simulink model "model_2022b"  (R2023b)
settings: Solver=VariableStepAuto  StartTime=0.0  StopTime=250  FixedStep=0.001  MaxStep=1e-2  RelTol=1e-3
undefined symbols (not defined in the file or in its folder): A, A0f, b, d, gamma, N, P
settings Model: Creator=Катя  LastModifiedBy=deniskirbaba

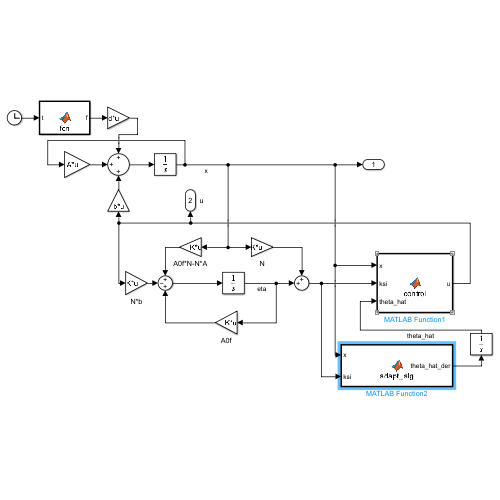
[thumbnail: Simulink's stored preview of the top-level diagram]
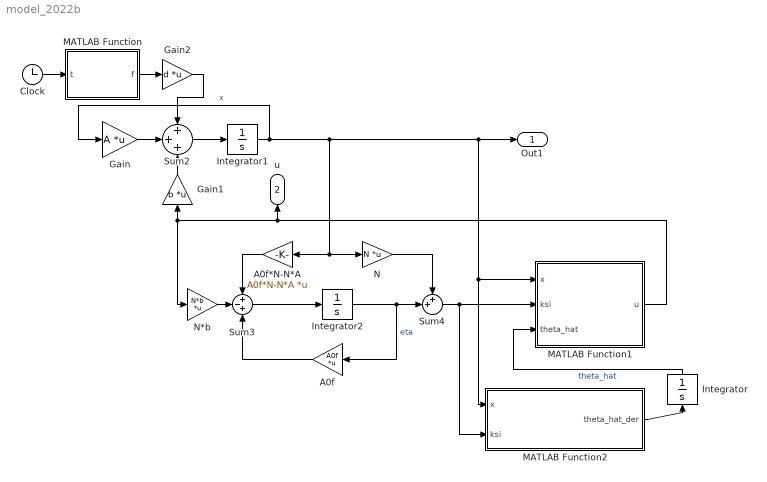
== system model_2022b ==
  A0f : Gain  Gain=A0f  Multiplication=Matrix(K*u)
  A0f*N-N*A : Gain  Gain=A0f*N-N*A  Multiplication=Matrix(K*u)
  Clock : Clock
  Gain : Gain  Gain=A  Multiplication=Matrix(K*u)
  Gain1 : Gain  Gain=b  Multiplication=Matrix(K*u)
  Gain2 : Gain  Gain=d  Multiplication=Matrix(K*u)
  Integrator : Integrator  InitialCondition=[0;0]
  Integrator1 : Integrator  InitialCondition=[0;0]
  Integrator2 : Integrator
  MATLAB Function : MATLAB Function  TreatAsAtomicUnit=on
  MATLAB Function1 : MATLAB Function  TreatAsAtomicUnit=on
  MATLAB Function2 : MATLAB Function  TreatAsAtomicUnit=on
  N : Gain  Gain=N  Multiplication=Matrix(K*u)
  N*b : Gain  Gain=N*b  Multiplication=Matrix(K*u)
  Sum2 : Sum  Inputs=+++
  Sum3 : Sum  Inputs=+-+
  Sum4 : Sum  Inputs=++|
  Out1 : Outport
  u : Outport  Port=2
  wires:
  Integrator1/1 -> Out1/1, MATLAB Function2/1(x), MATLAB Function1/1(x), N/1, A0f*N-N*A/1, Gain/1  "x"
  MATLAB Function2/1(theta_hat_der) -> Integrator/1
  Integrator/1 -> MATLAB Function1/3(theta_hat)  "theta_hat"
  Gain/1 -> Sum2/2
  Gain1/1 -> Sum2/3
  Sum2/1 -> Integrator1/1
  Gain2/1 -> Sum2/1
  Integrator2/1 -> A0f/1, Sum4/2  "eta"
  Sum3/1 -> Integrator2/1
  A0f/1 -> Sum3/3
  N*b/1 -> Sum3/2
  A0f*N-N*A/1 -> Sum3/1
  MATLAB Function1/1(u) -> u/1, N*b/1, Gain1/1
  N/1 -> Sum4/1
  Sum4/1 -> MATLAB Function2/2(ksi), MATLAB Function1/2(ksi)
  Clock/1 -> MATLAB Function/1(t)
  MATLAB Function/1(f) -> Gain2/1

== matlab function model_2022b/MATLAB Function1 ==
  data: x input; u output; ksi input; theta_hat input; K parameter
function u = control(x, ksi, theta_hat, K)
    u = -K*x-theta_hat.'*ksi;
end

== matlab function model_2022b/MATLAB Function ==
  data: t input; f output
function f = fcn(t)

f = 5*cos(5*t+1.5);

== matlab function model_2022b/MATLAB Function2 ==
  data: x input; ksi input; theta_hat_der output; gamma parameter; b parameter; P parameter
function theta_hat_der = adapt_alg(x, ksi, gamma, b, P)
    theta_hat_der = gamma * ksi * b.' * P * x;
end
